simulink model "ccm_basic_model"  (R2024b)
settings: Solver=ode23tb  StartTime=0.0  StopTime=0.3  MaxStep=5e-8  RelTol=1e-4
values from neighbouring files (symbols this model uses):
  C = 33e-6    (= 3.3e-05)    [MAIN_SCRIPT.m]
  L = 100e-6    (= 0.0001)    [MAIN_SCRIPT.m]
  P = ControllerDesign(P)    [MAIN_SCRIPT.m]
  R = 12    [MAIN_SCRIPT.m]
  Rc = 0.05    [MAIN_SCRIPT.m]
  Rl = 0.05    [MAIN_SCRIPT.m]
libraries: spsCurrentMeasurementLib x4, spsVoltageMeasurementLib x3, spsParallelRLCBranchLib x2, spsSeriesRLCBranchLib x2, spsBreakerLib x1, spsControlledVoltageSourceLib x1, spsDCVoltageSourceLib x1, spsDiodeLib x1, spsGroundLib x1, spsMeanLib x1, spsMosfetLib x1, spsSawtoothGeneratorLib x1
settings Model: Creator=S SURYA  LastModifiedBy=S SURYA
settings SolverCC: ZeroCrossAlgorithm=Adaptive
settings DebuggingCC: IgnoredZcDiagnostic=none

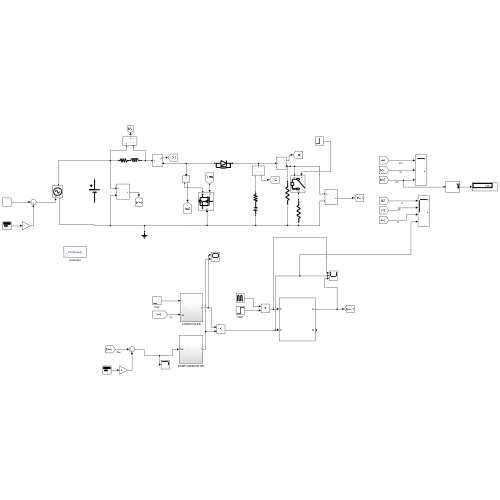
[thumbnail: Simulink's stored preview of the top-level diagram]
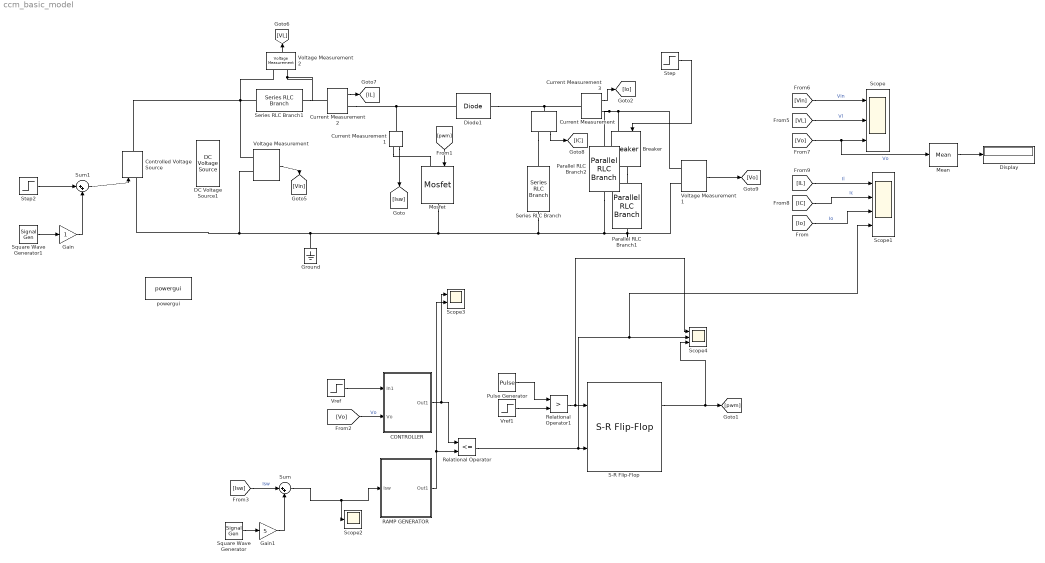
== system ccm_basic_model ==
  Breaker : spsBreakerLib/Breaker  InitialState=0  SwitchingTimes="[1/60  5/60]"  External=on  BreakerResistance=0.01  SnubberResistance=1e6  SnubberCapacitance=inf  Measurements=None  MoreParameters=on  NoBreakLoop=off
  "CONTROLLER " : Subsystem
  Controlled Voltage Source : spsControlledVoltageSourceLib/Controlled Voltage Source  Initialize=on  Source_Type=DC  Amplitude=0  Phase=0  Frequency=0  Measurements=None
  Current Measurement{,1..3} (4 alike) : spsCurrentMeasurementLib/Current Measurement  PhasorSimulation=off  OutputType=Complex  PSBequivalent=0
  DC Voltage Source1 : spsDCVoltageSourceLib/DC Voltage Source  Amplitude=P.Vi  Measurements=None
  Diode1 : spsDiodeLib/Diode  Ron=0.0001  Lon=0  Vf=0.8  IC=0  UseSnubber=0  Rs=500  Cs=250e-9  Measurements=off
  Display : Display
  Gain : Gain
  Gain1 : Gain  Gain=5
  Ground : spsGroundLib/Ground  LConnTagsString=a
  Mean : spsMeanLib/Mean  Freq=200e3  Vinit=0  Ts=0
  Mosfet : spsMosfetLib/Mosfet  Ron=0.1  Lon=0  Rd=0.01  Vfd=0  IC=0  Rs=1e5  Cs=inf  Measurements=off
  Parallel RLC Branch1 : spsParallelRLCBranchLib/Parallel RLC Branch  LConnTagsString=a  RConnTagsString=__new0  BranchType=R  Resistance=R*2  Inductance=200e-6  SetiL0=off  InitialCurrent=0  Capacitance=1e-6  Setx0=off  InitialVoltage=0  Measurements=None
  Parallel RLC Branch2 : spsParallelRLCBranchLib/Parallel RLC Branch  LConnTagsString=a  RConnTagsString=__new0  BranchType=R  Resistance=R  Inductance=200e-6  SetiL0=off  InitialCurrent=0  Capacitance=1e-6  Setx0=off  InitialVoltage=0  Measurements=None
  Pulse Generator : DiscretePulseGenerator  PulseType=Time based  Period=5e-6
  RAMP GENERATOR : Subsystem
  Relational Operator : RelationalOperator  Operator=<=  OutDataTypeStr=boolean  InputSameDT=off
  Relational Operator1 : RelationalOperator  Operator=>  OutDataTypeStr=boolean  InputSameDT=off
  S-R Flip-Flop : simulink_extras/Flip Flops/S-R Flip-Flop  initial_condition=0
  Scope : Scope  NumInputPorts=3
  Scope1 : Scope  NumInputPorts=4
  Scope2 : Scope
  Scope3 : Scope  NumInputPorts=2
  Scope4 : Scope  NumInputPorts=3
  Series RLC Branch : spsSeriesRLCBranchLib/Series RLC Branch  LConnTagsString=__new0  RConnTagsString=__new0  BranchType=RC  Resistance=Rc  Inductance=0  SetiL0=off  InitialCurrent=0  Capacitance=C  Setx0=off  InitialVoltage=0  Measurements=None
  Series RLC Branch1 : spsSeriesRLCBranchLib/Series RLC Branch  LConnTagsString=__new0  RConnTagsString=__new0  BranchType=RL  Resistance=Rl  Inductance=L  SetiL0=off  InitialCurrent=0  Capacitance=C  Setx0=off  InitialVoltage=0  Measurements=None
  Square Wave Generator : SignalGenerator  WaveForm=square  Amplitude=P.ILpeak*0.01  Frequency=100
  Square Wave Generator1 : SignalGenerator  WaveForm=square  Amplitude=P.Vi*0.01  Frequency=1000
  Step : Step  Time=0.15  SampleTime=0
  Step2 : Step  Time=0  After=P.Vi  SampleTime=0
  Sum : Sum  Inputs=|++
  Sum1 : Sum  Inputs=|++
  Voltage Measurement : spsVoltageMeasurementLib/Voltage Measurement  PhasorSimulation=off  OutputType=Complex  PSBequivalent=0
  Voltage Measurement1 : spsVoltageMeasurementLib/Voltage Measurement  PhasorSimulation=off  OutputType=Complex  PSBequivalent=0
  Voltage Measurement2 : spsVoltageMeasurementLib/Voltage Measurement  PhasorSimulation=off  OutputType=Complex  PSBequivalent=0
  Vref : Step  Time=0.25  Before=120  After=130  SampleTime=0
  Vref1 : Step  Time=0  After=0  SampleTime=0
  powergui : spspowerguiLib/powergui  Priority=1  SimulationMode=Continuous  SampleTime=1e-8  frequency=60  Iterations=50  frequencyindice=0  Pbase=100e6  ErrMax=1e-4  UnitsV=kV  UnitsW=MW  buscounter=0  FunctionMessages=off  echomessages=off  EnableUseOfTLC=off  CurrentSourceSwitches=off  DisableSnubberDevices=off  DisableRonSwitches=off  DisableVfSwitches=off  DisplayEquations=off  AutomaticDiscreteSolvers=off  SolverType=Tustin/Backward Euler (TBE)  Interpol=off  ExternalGateDelay=off  methode=off  Ts=100  x0status=blocks  SPID=on  SwTol=0  HookPort=off  NonlinearTolerance=1e-4  nMaxIteration=100  ContinueOnMaxIteration=off  RestoreLinks=warning  ResistiveCurrentMeasurement=off  Frange=[0:2:500]  Ylog=off  Xlog=on  ShowGrid=off  save=off  variable=ZData  structure=0  ZoomFFT=off  StartTime=0.0  cycles=1  DisplayStyle=1  fundamental=60  FreqAxis=off  MaxFrequency=1000  frequencyindicesteady=1  RmsSteady=1  display=off
  wires:
  Voltage Measurement2/1 -> [VL]
  [VL] -> Scope/2  "Vl"
  Current Measurement3/1 -> [Io]
  Current Measurement/1 -> [IC]
  [pwm] -> Mosfet/1
  [IL] -> Scope1/1  "Il"
  [Vin] -> Scope/1  "Vin"
  Current Measurement2/1 -> [IL]
  Voltage Measurement/1 -> [Vin]
  [Io] -> Scope1/3  "Io"
  [Vo] -> Mean/1, Scope/3  "Vo"
  [IC] -> Scope1/2  "Ic"
  Current Measurement1/1 -> [Isw]
  Mean/1 -> Display/1
  Step/1 -> Breaker/1
  [Isw] -> Sum/1  "Isw"
  Voltage Measurement1/1 -> [Vo]
  Vref/1 -> "CONTROLLER "/1(In1)
  [Vo] -> "CONTROLLER "/2(Vo)  "Vo"
  "CONTROLLER "/1(Out1) -> Scope3/1, Relational Operator/1
  RAMP GENERATOR/1(Out1) -> Scope3/2, Relational Operator/2
  S-R Flip-Flop/1 -> Scope4/3, [pwm]
  Relational Operator1/1 -> Scope4/1, S-R Flip-Flop/1
  Pulse Generator/1 -> Relational Operator1/1
  Vref1/1 -> Relational Operator1/2
  Relational Operator/1 -> Scope1/4, Scope4/2, S-R Flip-Flop/2
  Square Wave Generator/1 -> Gain1/1
  Sum/1 -> Scope2/1, RAMP GENERATOR/1(Isw)
  Sum1/1 -> Controlled Voltage Source/1
  Step2/1 -> Sum1/1
  Square Wave Generator1/1 -> Gain/1
  Gain1/1 -> Sum/2
  Gain/1 -> Sum1/2
  connections:
  Current Measurement2/RConn1 -- Current Measurement1/LConn1 -- Diode1/LConn1
  Parallel RLC Branch2/RConn1 -- Parallel RLC Branch1/RConn1 -- Voltage Measurement1/LConn2 -- Ground/LConn1 -- Voltage Measurement/LConn2 -- Controlled Voltage Source/LConn1 -- Mosfet/RConn1 -- Series RLC Branch/RConn1
  Voltage Measurement2/LConn2 -- Current Measurement2/LConn1 -- Series RLC Branch1/RConn1
  Voltage Measurement1/LConn1 -- Breaker/LConn1 -- Current Measurement3/RConn1 -- Parallel RLC Branch2/LConn1
  Current Measurement3/LConn1 -- Current Measurement/LConn1 -- Diode1/RConn1
  Voltage Measurement/LConn1 -- Controlled Voltage Source/RConn1 -- Series RLC Branch1/LConn1 -- Voltage Measurement2/LConn1
  Current Measurement1/RConn1 -- Mosfet/LConn1
  Current Measurement/RConn1 -- Series RLC Branch/LConn1
  Breaker/RConn1 -- Parallel RLC Branch1/LConn1

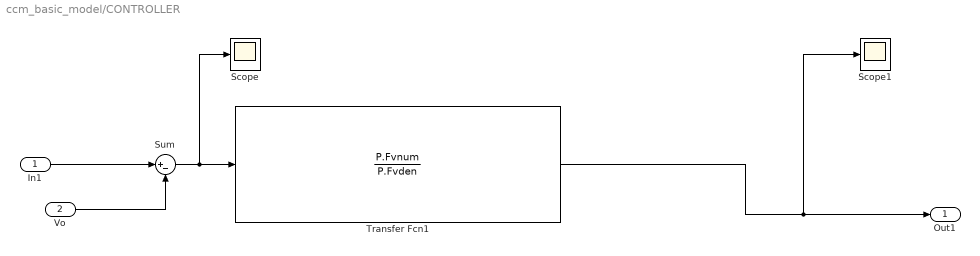
== system ccm_basic_model/CONTROLLER  ==
  In1 : Inport
  Vo : Inport  Port=2
  Scope : Scope
  Scope1 : Scope
  Sum : Sum  Inputs=|+-
  Transfer Fcn1 : TransferFcn  Numerator=P.Fvnum  Denominator=P.Fvden
  Out1 : Outport
  wires:
  Sum/1 -> Scope/1, Transfer Fcn1/1
  In1/1 -> Sum/1
  Vo/1 -> Sum/2
  Transfer Fcn1/1 -> Scope1/1, Out1/1

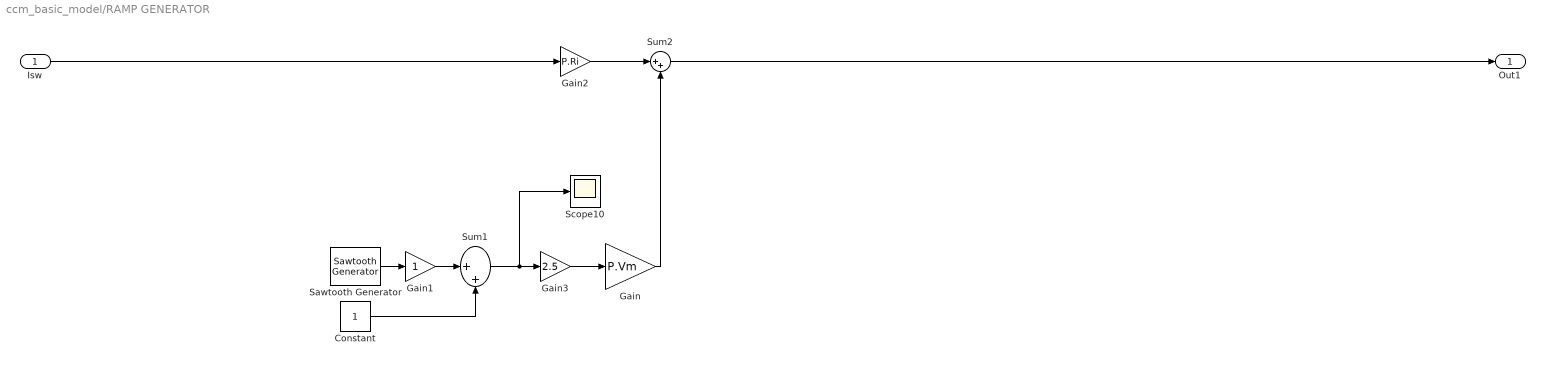
== system ccm_basic_model/RAMP GENERATOR ==
  Isw : Inport
  Constant : Constant
  Gain : Gain  Gain=P.Vm
  Gain1 : Gain
  Gain2 : Gain  Gain=P.Ri
  Gain3 : Gain  Gain=2.5
  Sawtooth Generator : spsSawtoothGeneratorLib/Sawtooth Generator  Freq=200e3  Phase=0  Ts=0
  Scope10 : Scope
  Sum1 : Sum  Inputs=|++
  Sum2 : Sum  Inputs=|++
  Out1 : Outport
  wires:
  Constant/1 -> Sum1/2
  Gain3/1 -> Gain/1
  Gain2/1 -> Sum2/1
  Sum1/1 -> Scope10/1, Gain3/1
  Sawtooth Generator/1 -> Gain1/1
  Sum2/1 -> Out1/1
  Gain/1 -> Sum2/2
  Gain1/1 -> Sum1/1
  Isw/1 -> Gain2/1
